simulink model "Modelo_Linear_Fase_2_Grupo_10"  (R2016a)
settings: Solver=VariableStepAuto  SolverMode=SingleTasking  StartTime=0.0  StopTime=20  RelTol=1e-3
values from neighbouring files (symbols this model uses):
  A_g = [0 0;1 0]    [Drone_Fase_2.m]
  A_lp = [0  0 0 0; 1 0 0 0; 0 -g 0 0; 0 0 1 0]    [Drone_Fase_2.m]
  A_lr = [0  0 0 0; 1 0 0 0; 0 g 0 0; 0 0 1 0]    [Drone_Fase_2.m]
  A_v = [0 0;1 0]    [Drone_Fase_2.m]
  B_g = [b_r;0]    [Drone_Fase_2.m]
  B_lp = [b_q;0;0;0]    [Drone_Fase_2.m]
  B_lr = [b_p;0;0;0]    [Drone_Fase_2.m]
  B_v = [-b_z ;0]    [Drone_Fase_2.m]
  C_g = [0  1]    [Drone_Fase_2.m]
  C_lp = [0 1 0 0; 0 0 0 1]    [Drone_Fase_2.m]
  C_lr = [0 1 0 0; 0 0 0 1]    [Drone_Fase_2.m]
  C_v = [0 1]    [Drone_Fase_2.m]
  Noise_g = [10^-6; 10^-1]    [Drone_Fase_2.m]
  Noise_lp = [10^-3; 0; Wind(1)/(m); 10^-1]    [Drone_Fase_2.m]
  Noise_lr = [10^-3; 0; Wind(2)/(m); 10^-1]    [Drone_Fase_2.m]
  Noise_v = [Wind(3)/(m); 1]    [Drone_Fase_2.m]
  var_pitch = 2.6060*10^(-4)    (= 0.0002606)    [Drone_Fase_2.m]
  var_px = 7.3221*10^(-4)    (= 0.00073221)    [Drone_Fase_2.m]
  var_py = 4.2829*10^(-4)    (= 0.00042829)    [Drone_Fase_2.m]
  var_pz = 1.8000*10^(-4)    (= 0.00018)    [Drone_Fase_2.m]
  var_roll = 3.4817*10^(-4)    (= 0.00034817)    [Drone_Fase_2.m]
  var_yaw = 3.8313*10^(-5)    (= 3.8313e-05)    [Drone_Fase_2.m]
undefined symbols (not defined in the file or in its folder): Lk_g, Lk_lp, Lk_lr, Lk_v, sigbuilder_block
libraries: simulink x8
settings Model: Creator=Ricardo Henriques  LastModifiedBy=Catarina
settings DebuggingCC: SFUnexpectedBacktrackingDiag=error  SFNoUnconditionalDefaultTransitionDiag=error
settings GRTTargetCC: TargetLangStandard=C99 (ISO)  GeneratePreprocessorConditionals=Use local settings
settings ConfigComp: CovMetricSettings=dwe  CovHtmlReporting=off  CovSaveCumulativeToWorkspaceVar=off  CovSaveSingleToWorkspaceVar=off  CovExternalEMLEnable=on

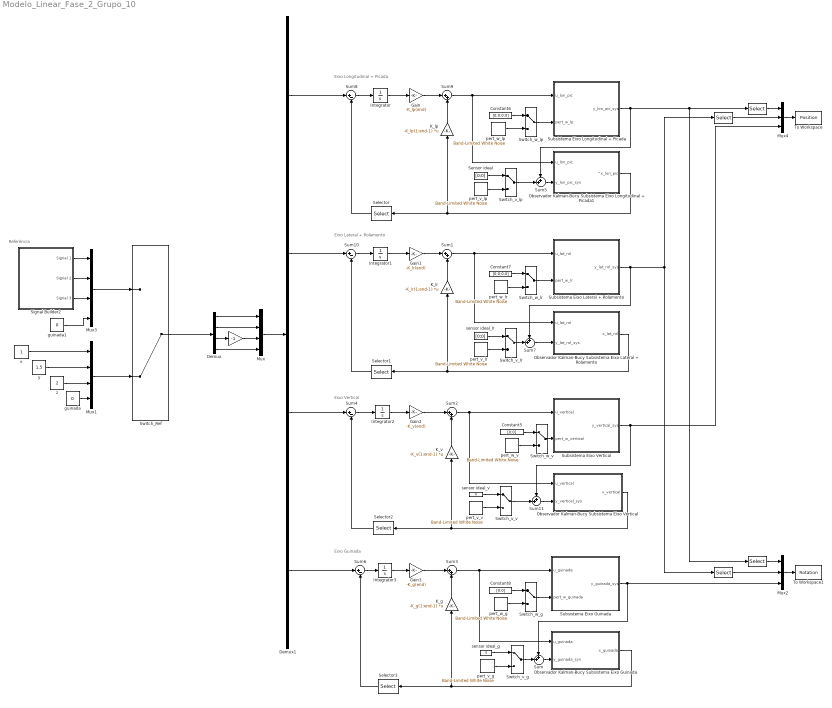
== system Modelo_Linear_Fase_2_Grupo_10 ==
  note: Eixo Guinada
  note: Eixo Vertical
  note: Eixo Lateral + Rolamento
  note: Eixo Longitudinal + Picada
  note: Referência
  " " : Selector  InputPortWidth=2  IndexOptions=Index vector (dialog)  Indices=[2]  OutputSizes=1
  "  " : Selector  InputPortWidth=2  IndexOptions=Index vector (dialog)  Indices=[1]  OutputSizes=1
  "    " : Selector  InputPortWidth=2  IndexOptions=Index vector (dialog)  Indices=[2]  OutputSizes=1
  "             " : Selector  InputPortWidth=2  IndexOptions=Index vector (dialog)  Indices=[1]  OutputSizes=1
  "                " : Gain  Gain=-1
  Constant5 : Constant  Value=[0;0]  VectorParams1D=off
  Constant6 : Constant  Value=[0;0;0;0]  VectorParams1D=off
  Constant7 : Constant  Value=[0;0;0;0]  VectorParams1D=off
  Constant8 : Constant  Value=[0;0]  VectorParams1D=off
  Demux : Demux
  Demux1 : Demux
  Gain : Gain  Gain=-K_lp(end)
  Gain1 : Gain  Gain=-K_lr(end)
  Gain2 : Gain  Gain=-K_v(end)
  Gain3 : Gain  Gain=-K_g(end)
  Integrator{,1..3} (4 alike) : Integrator
  K_g : Gain  Gain=-K_g(1:end-1)  Multiplication=Matrix(K*u) (u vector)
  K_lp : Gain  Gain=-K_lp(1:end-1)  Multiplication=Matrix(K*u) (u vector)
  K_lr : Gain  Gain=-K_lr(1:end-1)  Multiplication=Matrix(K*u) (u vector)
  K_v : Gain  Gain=-K_v(1:end-1)  Multiplication=Matrix(K*u) (u vector)
  Mux : Mux
  Mux1 : Mux
  Mux2 : Mux  Inputs=3
  Mux3 : Mux
  Mux4 : Mux  Inputs=3
  Observador Kalman-Bucy Subsistema Eixo Guinada : Subsystem
  Observador Kalman-Bucy Subsistema Eixo Lateral + Rolamento : Subsystem
  Observador Kalman-Bucy Subsistema Eixo Longitudinal + Picada1 : Subsystem
  Observador Kalman-Bucy Subsistema Eixo Vertical : Subsystem
  Selector : Selector  InputPortWidth=4  IndexOptions=Index vector (dialog)  Indices=[4]  OutputSizes=1
  Selector1 : Selector  InputPortWidth=4  IndexOptions=Index vector (dialog)  Indices=[4]  OutputSizes=1
  Selector2 : Selector  InputPortWidth=2  IndexOptions=Index vector (dialog)  Indices=[2]  OutputSizes=1
  Selector3 : Selector  InputPortWidth=2  IndexOptions=Index vector (dialog)  Indices=[2]  OutputSizes=1
  Sensor ideal : Constant  Value=[0;0]  VectorParams1D=off
  Signal Builder2 : Subsystem  Tag=STV Subsys  LoadFcn=sigbuilder_block('load');  StartFcn=sigbuilder_block('start');  StopFcn=sigbuilder_block('stop');  ClipboardFcn=sigbuilder_block('clipboard');  mask(Sigbuilder block){}
      mask help: Simulink:masks:SigbuilderBlock_MD
      mask init:
      | if ~strcmp(get_param(bdroot(gcbh),'SimulationStatus'),'stopped') tuvar = sigbuilder_block('maskInit'); end
      settings: CopyFcn=sigbuilder_block('copy');  DeleteFcn=sigbuilder_block('delete');  ModelCloseFcn=sigbuilder_block('modelClose');  PreSaveFcn=sigbuilder_block('preSave');  PauseFcn=sigbuilder_block('pause');  ContinueFcn=sigbuilder_block('continue');  NameChangeFcn=sigbuilder_block('namechange');  OpenFcn=sigbuilder_block('open',[208.2 56.4 858.6 509.4 ]);  CloseFcn=sigbuilder_block('close');
      mask Display: plot(0, 0, 100, 100,[2, 2, 32, 32, 2], [68, 8, 8, 68, 68],[32, 2], [38, 38], [32, 19, 2],[53, 60, 44], [32, 17, 17, 2],[16, 16, 31, 31]);txt = getActiveGroup(gcbh);text(2, 100, txt,'verticalAlignment', 'top');
  Subsistema Eixo Guinada : Subsystem
  Subsistema Eixo Lateral + Rolamento : Subsystem
  Subsistema Eixo Longitudinal + Picada : Subsystem
  Subsistema Eixo Vertical : Subsystem
  Sum{,5,7,11} (4 alike) : Sum  Inputs=++|
  Sum{1..3,9} (4 alike) : Sum  Inputs=|++
  Sum{4,6,8,10} (4 alike) : Sum  Inputs=|+-
  Switch_Ref : ManualSwitch  CurrentSetting=0
  Switch_v_g : ManualSwitch
  Switch_v_lp : ManualSwitch
  Switch_v_lr : ManualSwitch
  Switch_v_v : ManualSwitch
  Switch_w_g : ManualSwitch
  Switch_w_lp : ManualSwitch
  Switch_w_lr : ManualSwitch
  Switch_w_v : ManualSwitch
  To Workspace : ToWorkspace  VariableName=Position  SaveFormat=Timeseries  SampleTime=1/30
  To Workspace1 : ToWorkspace  VariableName=Rotation  SaveFormat=Timeseries  SampleTime=1/30
  guinada : Constant  Value=0
  guinada1 : Constant  Value=0
  pert_v_g : simulink/Sources/Band-Limited White Noise  Cov=var_yaw*0.005  Ts=0.005  seed=[23341]
  pert_v_lp : simulink/Sources/Band-Limited White Noise  Cov=[var_pitch*0.005; var_px*0.005]  Ts=0.005  seed=[23341]  VectorParams1D=off
  pert_v_lr : simulink/Sources/Band-Limited White Noise  Cov=[var_roll*0.005; var_py*0.005]  Ts=0.005  seed=[23341]  VectorParams1D=off
  pert_v_v : simulink/Sources/Band-Limited White Noise  Cov=var_pz*0.005  Ts=0.005  seed=[23341]  VectorParams1D=off
  pert_w_g : simulink/Sources/Band-Limited White Noise  Cov=Noise_g*0.005  Ts=0.005  seed=[23341]  VectorParams1D=off
  pert_w_lp : simulink/Sources/Band-Limited White Noise  Cov=Noise_lp*0.005  Ts=0.005  seed=[23341]  VectorParams1D=off
  pert_w_lr : simulink/Sources/Band-Limited White Noise  Cov=Noise_lr*0.005  Ts=0.005  seed=[23341]  VectorParams1D=off
  pert_w_v : simulink/Sources/Band-Limited White Noise  Cov=Noise_v*0.005  Ts=0.005  seed=[23341]  VectorParams1D=off
  sensor ideal_g : Constant  Value=0  VectorParams1D=off
  sensor ideal_lr : Constant  Value=[0;0]  VectorParams1D=off
  sensor ideal_v : Constant  Value=0  VectorParams1D=off
  x : Constant
  y : Constant  Value=1.5
  z : Constant  Value=2
  wires:
  Observador Kalman-Bucy Subsistema Eixo Longitudinal + Picada1/1(^x_lon_pic) -> K_lp/1, Selector/1
  K_lp/1 -> Sum9/2
  Subsistema Eixo Longitudinal + Picada/1("y_lon_pic_sys ") -> Sum5/1, "  "/1, " "/1
  Observador Kalman-Bucy Subsistema Eixo Lateral + Rolamento/1(x_lat_rol) -> Selector1/1, K_lr/1
  K_lr/1 -> Sum1/2
  Subsistema Eixo Vertical/1("y_vertical_sys ") -> Sum11/1, Mux4/3
  Observador Kalman-Bucy Subsistema Eixo Vertical/1(x_vertical) -> K_v/1, Selector2/1
  K_v/1 -> Sum2/2
  K_g/1 -> Sum3/2
  Observador Kalman-Bucy Subsistema Eixo Guinada/1(x_guinada) -> K_g/1, Selector3/1
  Subsistema Eixo Guinada/1("y_guinada_sys ") -> Sum/1, Mux2/3
  Demux1/4 -> Sum6/1
  Demux1/2 -> Sum10/1
  Demux1/1 -> Sum8/1
  Sum8/1 -> Integrator/1
  Sum10/1 -> Integrator1/1
  Sum4/1 -> Integrator2/1
  Sum6/1 -> Integrator3/1
  Integrator/1 -> Gain/1
  Integrator1/1 -> Gain1/1
  Integrator2/1 -> Gain2/1
  Integrator3/1 -> Gain3/1
  Gain/1 -> Sum9/1
  Gain1/1 -> Sum1/1
  Gain2/1 -> Sum2/1
  Gain3/1 -> Sum3/1
  Sum2/1 -> Observador Kalman-Bucy Subsistema Eixo Vertical/1(u_vertical), Subsistema Eixo Vertical/1(u_vertical)
  Subsistema Eixo Lateral + Rolamento/1("y_lat_rol_sys ") -> Sum7/1, "             "/1, "    "/1
  pert_v_lp/1 -> Switch_v_lp/2
  pert_v_lr/1 -> Switch_v_lr/2
  pert_v_v/1 -> Switch_v_v/2
  pert_v_g/1 -> Switch_v_g/2
  Sensor ideal/1 -> Switch_v_lp/1
  sensor ideal_lr/1 -> Switch_v_lr/1
  sensor ideal_v/1 -> Switch_v_v/1
  sensor ideal_g/1 -> Switch_v_g/1
  Mux2/1 -> To Workspace1/1
  Mux4/1 -> To Workspace/1
  Switch_w_v/1 -> Subsistema Eixo Vertical/2(pert_w_vertical)
  pert_w_v/1 -> Switch_w_v/2
  Constant5/1 -> Switch_w_v/1
  Constant6/1 -> Switch_w_lp/1
  Switch_w_lp/1 -> Subsistema Eixo Longitudinal + Picada/2(pert_w_lp)
  pert_w_lp/1 -> Switch_w_lp/2
  Constant7/1 -> Switch_w_lr/1
  Switch_w_lr/1 -> Subsistema Eixo Lateral + Rolamento/2(pert_w_lr)
  pert_w_lr/1 -> Switch_w_lr/2
  Constant8/1 -> Switch_w_g/1
  Switch_w_g/1 -> Subsistema Eixo Guinada/2(pert_w_guinada)
  pert_w_g/1 -> Switch_w_g/2
  Sum5/1 -> Observador Kalman-Bucy Subsistema Eixo Longitudinal + Picada1/2("y_lon_pic_sys ")
  Switch_v_lp/1 -> Sum5/2
  Sum7/1 -> Observador Kalman-Bucy Subsistema Eixo Lateral + Rolamento/2("y_lat_rol_sys ")
  Switch_v_lr/1 -> Sum7/2
  Sum11/1 -> Observador Kalman-Bucy Subsistema Eixo Vertical/2("y_vertical_sys ")
  Switch_v_v/1 -> Sum11/2
  Selector/1 -> Sum8/2
  Selector1/1 -> Sum10/2
  Selector2/1 -> Sum4/2
  Sum/1 -> Observador Kalman-Bucy Subsistema Eixo Guinada/2("y_guinada_sys ")
  Switch_v_g/1 -> Sum/2
  Selector3/1 -> Sum6/2
  " "/1 -> Mux4/1
  "    "/1 -> Mux4/2
  "  "/1 -> Mux2/1
  "             "/1 -> Mux2/2
  Demux/3 -> "                "/1
  "                "/1 -> Mux/3
  Demux/4 -> Mux/4
  Demux/2 -> Mux/2
  Demux/1 -> Mux/1
  Mux/1 -> Demux1/1
  Mux1/1 -> Switch_Ref/2
  Mux3/1 -> Switch_Ref/1
  x/1 -> Mux1/1
  y/1 -> Mux1/2
  guinada/1 -> Mux1/4
  z/1 -> Mux1/3
  guinada1/1 -> Mux3/4
  Signal Builder2/1(Signal 1) -> Mux3/1
  Signal Builder2/2(Signal 2) -> Mux3/2
  Signal Builder2/3(Signal 3) -> Mux3/3
  Switch_Ref/1 -> Demux/1
  Demux1/3 -> Sum4/1
  Sum3/1 -> Subsistema Eixo Guinada/1(u_guinada), Observador Kalman-Bucy Subsistema Eixo Guinada/1(u_guinada)
  Sum1/1 -> Observador Kalman-Bucy Subsistema Eixo Lateral + Rolamento/1(u_lat_rol), Subsistema Eixo Lateral + Rolamento/1(u_lat_rol)
  Sum9/1 -> Observador Kalman-Bucy Subsistema Eixo Longitudinal + Picada1/1(u_lon_pic), Subsistema Eixo Longitudinal + Picada/1(u_lon_pic)

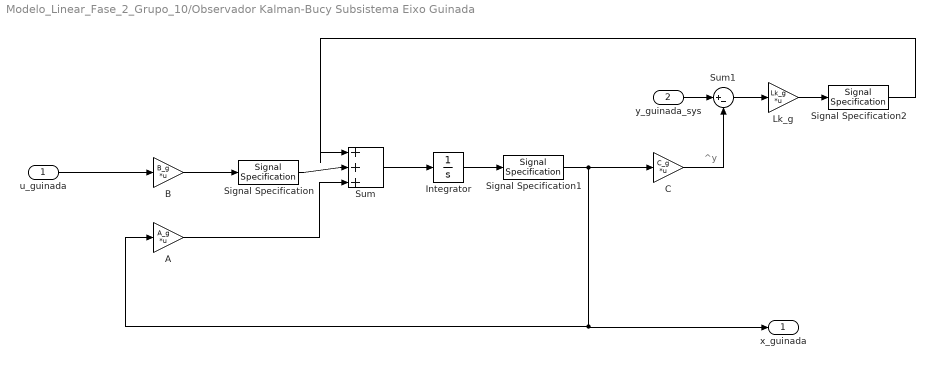
== system Modelo_Linear_Fase_2_Grupo_10/Observador Kalman-Bucy Subsistema Eixo Guinada ==
  note: ^y
  u_guinada : Inport
  "y_guinada_sys " : Inport  Port=2
  A : Gain  Gain=A_g  Multiplication=Matrix(K*u)
  B : Gain  Gain=B_g  Multiplication=Matrix(K*u)
  C : Gain  Gain=C_g  Multiplication=Matrix(K*u)
  Integrator : Integrator  InitialCondition=[0;0]
  Lk_g : Gain  Gain=Lk_g  Multiplication=Matrix(K*u) (u vector)
  Signal Specification : SignalSpecification  Dimensions=[2 1]
  Signal Specification1 : SignalSpecification  Dimensions=[2 1]
  Signal Specification2 : SignalSpecification  Dimensions=[2 1]
  Sum : Sum  Inputs=|+++
  Sum1 : Sum  Inputs=|+-
  x_guinada : Outport
  wires:
  B/1 -> Signal Specification/1
  Sum/1 -> Integrator/1
  Integrator/1 -> Signal Specification1/1
  A/1 -> Sum/3
  Signal Specification1/1 -> x_guinada/1, A/1, C/1
  u_guinada/1 -> B/1
  C/1 -> Sum1/2
  Signal Specification/1 -> Sum/2
  "y_guinada_sys "/1 -> Sum1/1
  Sum1/1 -> Lk_g/1
  Lk_g/1 -> Signal Specification2/1
  Signal Specification2/1 -> Sum/1

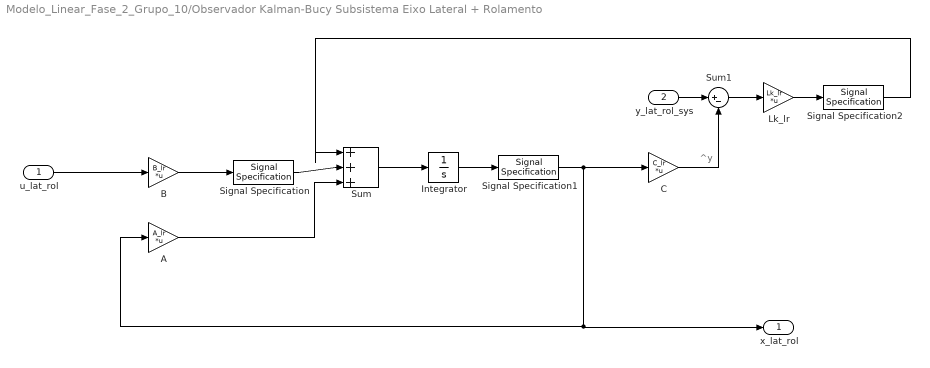
== system Modelo_Linear_Fase_2_Grupo_10/Observador Kalman-Bucy Subsistema Eixo Lateral + Rolamento ==
  note: ^y
  u_lat_rol : Inport
  "y_lat_rol_sys " : Inport  Port=2
  A : Gain  Gain=A_lr  Multiplication=Matrix(K*u)
  B : Gain  Gain=B_lr  Multiplication=Matrix(K*u)
  C : Gain  Gain=C_lr  Multiplication=Matrix(K*u)
  Integrator : Integrator  InitialCondition=[0;0;0;0]
  Lk_lr : Gain  Gain=Lk_lr  Multiplication=Matrix(K*u) (u vector)
  Signal Specification : SignalSpecification  Dimensions=[4 1]
  Signal Specification1 : SignalSpecification  Dimensions=[4 1]
  Signal Specification2 : SignalSpecification  Dimensions=[4 1]
  Sum : Sum  Inputs=|+++
  Sum1 : Sum  Inputs=|+-
  x_lat_rol : Outport
  wires:
  B/1 -> Signal Specification/1
  Sum/1 -> Integrator/1
  Integrator/1 -> Signal Specification1/1
  A/1 -> Sum/3
  Signal Specification1/1 -> x_lat_rol/1, A/1, C/1
  u_lat_rol/1 -> B/1
  C/1 -> Sum1/2
  Signal Specification/1 -> Sum/2
  "y_lat_rol_sys "/1 -> Sum1/1
  Sum1/1 -> Lk_lr/1
  Lk_lr/1 -> Signal Specification2/1
  Signal Specification2/1 -> Sum/1

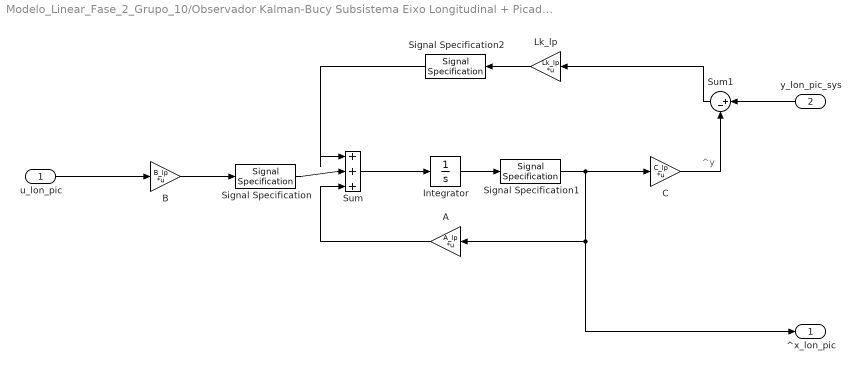
== system Modelo_Linear_Fase_2_Grupo_10/Observador Kalman-Bucy Subsistema Eixo Longitudinal + Picada1 ==
  note: ^y
  u_lon_pic : Inport
  "y_lon_pic_sys " : Inport  Port=2
  A : Gain  Gain=A_lp  Multiplication=Matrix(K*u)
  B : Gain  Gain=B_lp  Multiplication=Matrix(K*u)
  C : Gain  Gain=C_lp  Multiplication=Matrix(K*u)
  Integrator : Integrator  InitialCondition=[0;0;0;0]
  Lk_lp : Gain  Gain=Lk_lp  Multiplication=Matrix(K*u) (u vector)
  Signal Specification : SignalSpecification  Dimensions=[4 1]
  Signal Specification1 : SignalSpecification  Dimensions=[4 1]
  Signal Specification2 : SignalSpecification  Dimensions=[4 1]
  Sum : Sum  Inputs=|+++
  Sum1 : Sum  Inputs=|+-
  ^x_lon_pic : Outport
  wires:
  B/1 -> Signal Specification/1
  Sum/1 -> Integrator/1
  Integrator/1 -> Signal Specification1/1
  A/1 -> Sum/3
  Signal Specification1/1 -> ^x_lon_pic/1, A/1, C/1
  u_lon_pic/1 -> B/1
  C/1 -> Sum1/2
  Signal Specification/1 -> Sum/2
  "y_lon_pic_sys "/1 -> Sum1/1
  Sum1/1 -> Lk_lp/1
  Lk_lp/1 -> Signal Specification2/1
  Signal Specification2/1 -> Sum/1

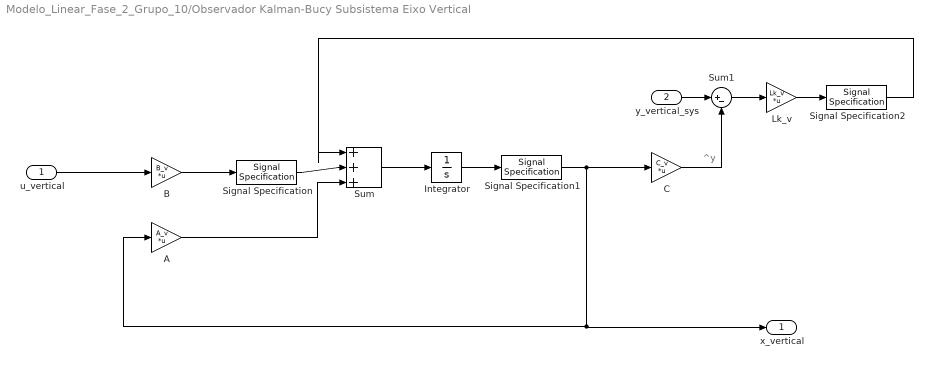
== system Modelo_Linear_Fase_2_Grupo_10/Observador Kalman-Bucy Subsistema Eixo Vertical ==
  note: ^y
  u_vertical : Inport
  "y_vertical_sys " : Inport  Port=2
  A : Gain  Gain=A_v  Multiplication=Matrix(K*u)
  B : Gain  Gain=B_v  Multiplication=Matrix(K*u)
  C : Gain  Gain=C_v  Multiplication=Matrix(K*u)
  Integrator : Integrator  InitialCondition=[0;0]
  Lk_v : Gain  Gain=Lk_v  Multiplication=Matrix(K*u) (u vector)
  Signal Specification : SignalSpecification  Dimensions=[2 1]
  Signal Specification1 : SignalSpecification  Dimensions=[2 1]
  Signal Specification2 : SignalSpecification  Dimensions=[2 1]
  Sum : Sum  Inputs=|+++
  Sum1 : Sum  Inputs=|+-
  x_vertical : Outport
  wires:
  B/1 -> Signal Specification/1
  Sum/1 -> Integrator/1
  Integrator/1 -> Signal Specification1/1
  A/1 -> Sum/3
  Signal Specification1/1 -> x_vertical/1, A/1, C/1
  u_vertical/1 -> B/1
  C/1 -> Sum1/2
  Signal Specification/1 -> Sum/2
  "y_vertical_sys "/1 -> Sum1/1
  Sum1/1 -> Lk_v/1
  Lk_v/1 -> Signal Specification2/1
  Signal Specification2/1 -> Sum/1

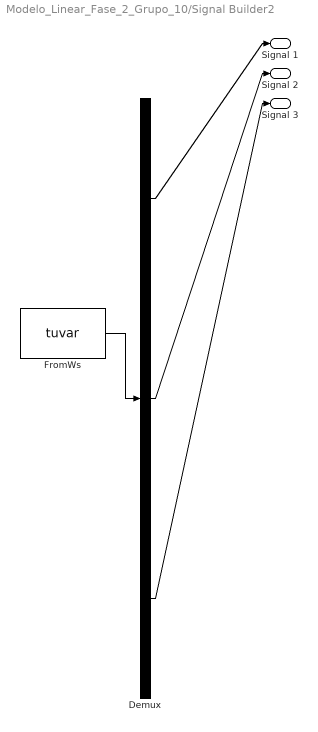
== system Modelo_Linear_Fase_2_Grupo_10/Signal Builder2 ==
  Demux : Demux  Tag=STV Demux  Outputs=3
  FromWs : FromWorkspace  Tag=STV FromWs  VariableName=tuvar  SampleTime=0
      SigBuilderData=|
      | common.afterFinalStr = 'Extrapolate'
      | common.sampleTime = 0
      | dataSet.timeRange = [0 60]
      | dataSet.name = 'Group 1'
      | sbobj.Groups.Name = 'Group 1'
      | sbobj.Groups.Signals(1).Name = 'Signal 1'
      | sbobj.Groups.Signals(1).XData = [0 1 2 3 4 5 6 7 8 9 10 10 11 12 13 14 15 16 17 18 19 20 21 22 23 24 25 26 27 28 29 30 31 32 33 34 35 36 37 38 39 40 41 42 43 44 45 46 47 48 49 50 51 52 53 54 55 56 57 58 59 60]
      | sbobj.Groups.Signals(1).YData = [0 0 0 0 0 0 0 0 2 2 1.98 2 2 2 2 2 2 2 2 2 2 -2 -2 -2 -2 -2 -2 -2 -2 2 2 2 2 2 2 2 2 2 2 2 2 -2 -2 -2 -2 -2 -2 -2 -2 -2 -2 2 2 2 2 2 2 2 0 0 0 0]
      | sbobj.Groups.Signals(2).Name = 'Signal 2'
      | sbobj.Groups.Signals(2).XData = [0 1 2 3 4 4 5 6 7 8 9 10 11 12 13 14 15 16 17 18 19 20 21 22 23 24 25 26 27 28 29 30 31 32 33 34 35 36 37 38 39 40 41 42 43 44 45 46 47 48 49 50 51 52 53 54 55 56 57 58 59 60]
      | sbobj.Groups.Signals(2).YData = [0 2 2 2 1.98 2 2 2 2 -2 -2 -2 -2 -2 -2 -2 -2 -2 -2 -2 -2 2 2 2 2 2 2 2 2 2 2 2 2 -2 -2 -2 -2 -2 -2 -2 -2 -2 -2 -2 -2 2 2 2 2 2 2 2 2 2 2 2 2 -2 -2 -1.95 -2 -2]
      | sbobj.Groups.Signals(3).Name = 'Signal 3'
      | sbobj.Groups.Signals(3).XData = [0 24 36 55 60]
      | sbobj.Groups.Signals(3).YData = [0 1 1 0 0]
      | sbobj.Groups.TimeRange = [0 60]
  Signal 1 : Outport  Tag=STV Outport
  Signal 2 : Outport  Tag=STV Outport  Port=2
  Signal 3 : Outport  Tag=STV Outport  Port=3
  wires:
  FromWs/1 -> Demux/1
  Demux/1 -> Signal 1/1
  Demux/2 -> Signal 2/1
  Demux/3 -> Signal 3/1

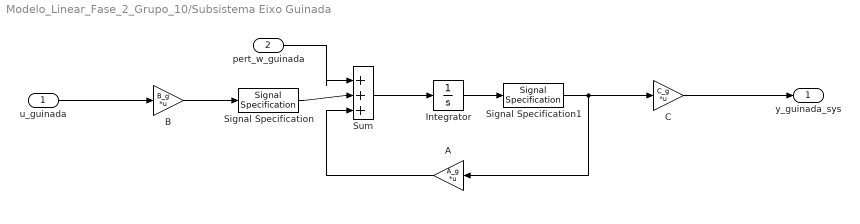
== system Modelo_Linear_Fase_2_Grupo_10/Subsistema Eixo Guinada ==
  u_guinada : Inport
  pert_w_guinada : Inport  Port=2
  A : Gain  Gain=A_g  Multiplication=Matrix(K*u)
  B : Gain  Gain=B_g  Multiplication=Matrix(K*u)
  C : Gain  Gain=C_g  Multiplication=Matrix(K*u)
  Integrator : Integrator  InitialCondition=[0;0]
  Signal Specification : SignalSpecification  Dimensions=[2 1]
  Signal Specification1 : SignalSpecification  Dimensions=[2 1]
  Sum : Sum  Inputs=|+++
  "y_guinada_sys " : Outport
  wires:
  B/1 -> Signal Specification/1
  Sum/1 -> Integrator/1
  Integrator/1 -> Signal Specification1/1
  Signal Specification1/1 -> C/1, A/1
  u_guinada/1 -> B/1
  C/1 -> "y_guinada_sys "/1
  A/1 -> Sum/3
  Signal Specification/1 -> Sum/2
  pert_w_guinada/1 -> Sum/1

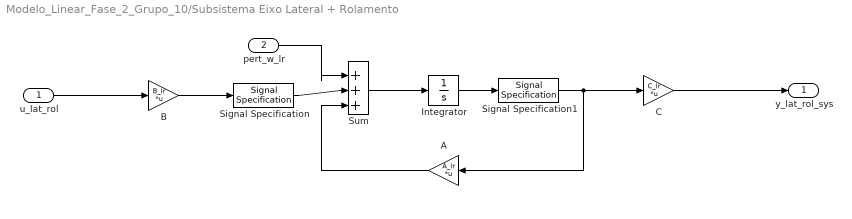
== system Modelo_Linear_Fase_2_Grupo_10/Subsistema Eixo Lateral + Rolamento ==
  u_lat_rol : Inport
  pert_w_lr : Inport  Port=2
  A : Gain  Gain=A_lr  Multiplication=Matrix(K*u)
  B : Gain  Gain=B_lr  Multiplication=Matrix(K*u)
  C : Gain  Gain=C_lr  Multiplication=Matrix(K*u)
  Integrator : Integrator  InitialCondition=[0;0;0;0]
  Signal Specification : SignalSpecification  Dimensions=[4 1]
  Signal Specification1 : SignalSpecification  Dimensions=[4 1]
  Sum : Sum  Inputs=|+++
  "y_lat_rol_sys " : Outport
  wires:
  B/1 -> Signal Specification/1
  Sum/1 -> Integrator/1
  Integrator/1 -> Signal Specification1/1
  Signal Specification1/1 -> C/1, A/1
  u_lat_rol/1 -> B/1
  C/1 -> "y_lat_rol_sys "/1
  A/1 -> Sum/3
  Signal Specification/1 -> Sum/2
  pert_w_lr/1 -> Sum/1

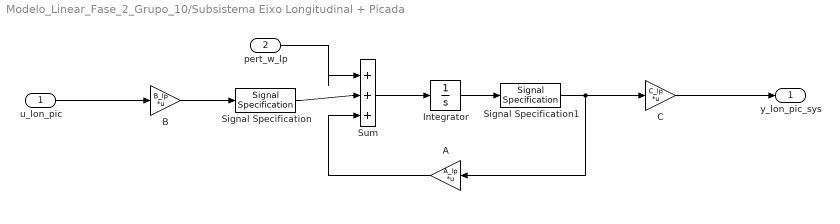
== system Modelo_Linear_Fase_2_Grupo_10/Subsistema Eixo Longitudinal + Picada ==
  u_lon_pic : Inport
  pert_w_lp : Inport  Port=2
  A : Gain  Gain=A_lp  Multiplication=Matrix(K*u)
  B : Gain  Gain=B_lp  Multiplication=Matrix(K*u)
  C : Gain  Gain=C_lp  Multiplication=Matrix(K*u)
  Integrator : Integrator  InitialCondition=[0;0;0;0]  ZeroCross=off
  Signal Specification : SignalSpecification  Dimensions=[4 1]
  Signal Specification1 : SignalSpecification  Dimensions=[4 1]
  Sum : Sum  Inputs=|+++
  "y_lon_pic_sys " : Outport
  wires:
  B/1 -> Signal Specification/1
  Sum/1 -> Integrator/1
  Integrator/1 -> Signal Specification1/1
  Signal Specification1/1 -> C/1, A/1
  u_lon_pic/1 -> B/1
  C/1 -> "y_lon_pic_sys "/1
  Signal Specification/1 -> Sum/2
  pert_w_lp/1 -> Sum/1
  A/1 -> Sum/3

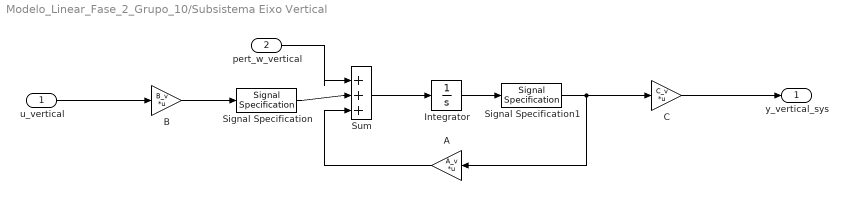
== system Modelo_Linear_Fase_2_Grupo_10/Subsistema Eixo Vertical ==
  u_vertical : Inport
  pert_w_vertical : Inport  Port=2
  A : Gain  Gain=A_v  Multiplication=Matrix(K*u)
  B : Gain  Gain=B_v  Multiplication=Matrix(K*u)
  C : Gain  Gain=C_v  Multiplication=Matrix(K*u)
  Integrator : Integrator  InitialCondition=[0;0]
  Signal Specification : SignalSpecification  Dimensions=[2 1]
  Signal Specification1 : SignalSpecification  Dimensions=[2 1]
  Sum : Sum  Inputs=|+++
  "y_vertical_sys " : Outport
  wires:
  B/1 -> Signal Specification/1
  Sum/1 -> Integrator/1
  Integrator/1 -> Signal Specification1/1
  Signal Specification1/1 -> C/1, A/1
  u_vertical/1 -> B/1
  C/1 -> "y_vertical_sys "/1
  A/1 -> Sum/3
  Signal Specification/1 -> Sum/2
  pert_w_vertical/1 -> Sum/1
